simulink model "HighLevel_Example"  (R2024a)
settings: Solver=VariableStepAuto  StartTime=0.0  StopTime=10.0  RelTol=1e-3
settings Model: Creator=Tamir Azaouag  LastModifiedBy=Tamir Azaouag

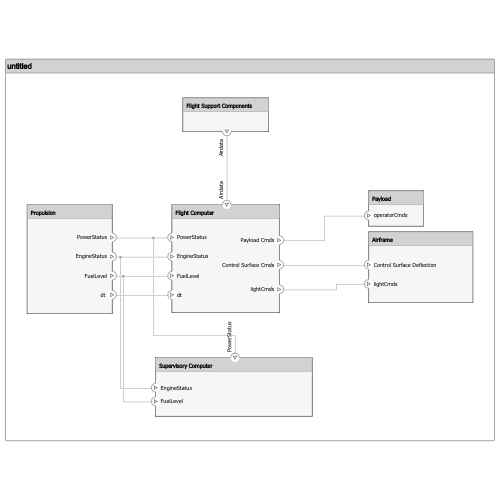
[thumbnail: Simulink's stored preview of the top-level diagram]
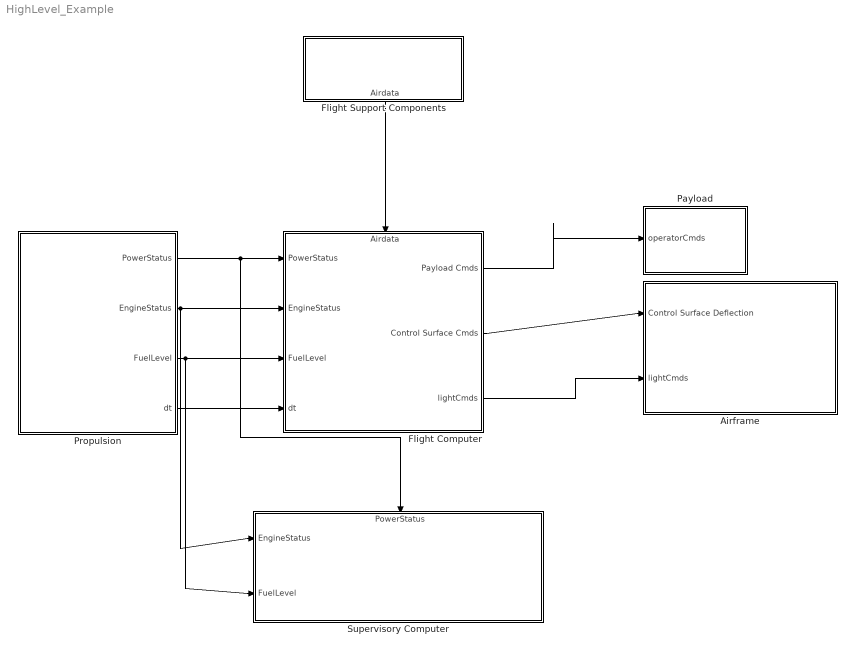
== system HighLevel_Example ==
  Airframe : Subsystem
      settings: PortSchema="{\"entries\":[{\"content\":{\"headerSize\":26,\"margin\":15,\"minimumSpacing\":25,\"sides\":[{\"content\":{\"connectorIds\":[\"In1\",\"In2\"]},\"type\":\"ConnectorPlacement.EquallySpacedRectSide\",\"uuid\":\"2c5e2d04-4906-4331-9418-21fa8db35aaf\"},{\"content\":{\"side\":\"RIGHT\"},\"type\":\"ConnectorPlacement.EquallySpacedRectSide\",\"uuid\":\"94a89f28-0e32-42bb-af58-158d3f1cfd39\"},{\"content\":{\"side\":\"TOP\"},\"type\":\"ConnectorPlacement.EquallySpacedRectSide\",\"uuid\":\"d206ce3f-8f92-44db-9478-82f14b2d4cfb\"}]},\"type\":\"ConnectorPlacement.EquallySpacedConnector\",\"uuid\":\"3d641880-63ee-42e2-927a-a7c9f20600aa\"}],\"packageUris\":[\"http://schema.mathworks.com/mf0/Connector/R2020b\"],\"version\":\"1.0\"}"
  Flight Computer : Subsystem
      settings: PortSchema="{\"entries\":[{\"content\":{\"headerSize\":26,\"margin\":15,\"minimumSpacing\":25,\"sides\":[{\"content\":{\"connectorIds\":[\"In1\",\"In2\",\"In3\",\"In4\"]},\"type\":\"ConnectorPlacement.EquallySpacedRectSide\",\"uuid\":\"2c5e2d04-4906-4331-9418-21fa8db35aaf\"},{\"content\":{\"connectorIds\":[\"Out1\",\"Out2\",\"Out3\"],\"side\":\"RIGHT\"},\"type\":\"ConnectorPlacement.EquallySpacedRectSide\",\"uuid\":\"94a89f28-0e32-42bb-af58-158d3f1cfd39\"},{\"content\":{\"connectorIds\":[\"In5\"],\"side\":\"TOP\"},\"type\":\"ConnectorPlacement.EquallySpacedRectSide\",\"uuid\":\"d206ce3f-8f92-44db-9478-82f14b2d4cfb\"}]},\"type\":\"ConnectorPlacement.EquallySpacedConnector\",\"uuid\":\"3d641880-63ee-42e2-927a-a7c9f20600aa\"}],\"packageUris\":[\"http://schema.mathworks.com/mf0/Connector/R2020b\"],\"version\":\"1.0\"}"
  Flight Support Components : Subsystem
      settings: PortSchema="{\"entries\":[{\"content\":{\"headerSize\":26,\"margin\":15,\"minimumSpacing\":25,\"sides\":[{\"content\":{},\"type\":\"ConnectorPlacement.EquallySpacedRectSide\",\"uuid\":\"2c5e2d04-4906-4331-9418-21fa8db35aaf\"},{\"content\":{\"side\":\"RIGHT\"},\"type\":\"ConnectorPlacement.EquallySpacedRectSide\",\"uuid\":\"94a89f28-0e32-42bb-af58-158d3f1cfd39\"},{\"content\":{\"side\":\"TOP\"},\"type\":\"ConnectorPlacement.EquallySpacedRectSide\",\"uuid\":\"d206ce3f-8f92-44db-9478-82f14b2d4cfb\"},{\"content\":{\"connectorIds\":[\"Out1\"],\"side\":\"BOTTOM\"},\"type\":\"ConnectorPlacement.EquallySpacedRectSide\",\"uuid\":\"ce0da822-1c1c-451b-a130-825bfb22f620\"}]},\"type\":\"ConnectorPlacement.EquallySpacedConnector\",\"uuid\":\"3d641880-63ee-42e2-927a-a7c9f20600aa\"}],\"packageUris\":[\"http://schema.mathworks.com/mf0/Connector/R2020b\"],\"version\":\"1.0\"}"
  "Payload " : Subsystem
      settings: PortSchema="{\"entries\":[{\"content\":{\"headerSize\":26,\"margin\":15,\"minimumSpacing\":25,\"sides\":[{\"content\":{\"connectorIds\":[\"In1\"]},\"type\":\"ConnectorPlacement.EquallySpacedRectSide\",\"uuid\":\"2c5e2d04-4906-4331-9418-21fa8db35aaf\"},{\"content\":{\"side\":\"RIGHT\"},\"type\":\"ConnectorPlacement.EquallySpacedRectSide\",\"uuid\":\"94a89f28-0e32-42bb-af58-158d3f1cfd39\"},{\"content\":{\"side\":\"TOP\"},\"type\":\"ConnectorPlacement.EquallySpacedRectSide\",\"uuid\":\"d206ce3f-8f92-44db-9478-82f14b2d4cfb\"}]},\"type\":\"ConnectorPlacement.EquallySpacedConnector\",\"uuid\":\"3d641880-63ee-42e2-927a-a7c9f20600aa\"}],\"packageUris\":[\"http://schema.mathworks.com/mf0/Connector/R2020b\"],\"version\":\"1.0\"}"
  "Propulsion " : Subsystem
      settings: PortSchema="{\"entries\":[{\"content\":{\"headerSize\":26,\"margin\":15,\"minimumSpacing\":25,\"sides\":[{\"content\":{},\"type\":\"ConnectorPlacement.EquallySpacedRectSide\",\"uuid\":\"2c5e2d04-4906-4331-9418-21fa8db35aaf\"},{\"content\":{\"connectorIds\":[\"Out1\",\"Out2\",\"Out3\",\"Out4\"],\"side\":\"RIGHT\"},\"type\":\"ConnectorPlacement.EquallySpacedRectSide\",\"uuid\":\"94a89f28-0e32-42bb-af58-158d3f1cfd39\"},{\"content\":{\"side\":\"TOP\"},\"type\":\"ConnectorPlacement.EquallySpacedRectSide\",\"uuid\":\"d206ce3f-8f92-44db-9478-82f14b2d4cfb\"}]},\"type\":\"ConnectorPlacement.EquallySpacedConnector\",\"uuid\":\"3d641880-63ee-42e2-927a-a7c9f20600aa\"}],\"packageUris\":[\"http://schema.mathworks.com/mf0/Connector/R2020b\"],\"version\":\"1.0\"}"
  Supervisory Computer : Subsystem
      settings: PortSchema="{\"entries\":[{\"content\":{\"headerSize\":26,\"margin\":15,\"minimumSpacing\":25,\"sides\":[{\"content\":{\"connectorIds\":[\"In1\",\"In2\"]},\"type\":\"ConnectorPlacement.EquallySpacedRectSide\",\"uuid\":\"2c5e2d04-4906-4331-9418-21fa8db35aaf\"},{\"content\":{\"side\":\"RIGHT\"},\"type\":\"ConnectorPlacement.EquallySpacedRectSide\",\"uuid\":\"94a89f28-0e32-42bb-af58-158d3f1cfd39\"},{\"content\":{\"connectorIds\":[\"In3\"],\"side\":\"TOP\"},\"type\":\"ConnectorPlacement.EquallySpacedRectSide\",\"uuid\":\"d206ce3f-8f92-44db-9478-82f14b2d4cfb\"}]},\"type\":\"ConnectorPlacement.EquallySpacedConnector\",\"uuid\":\"3d641880-63ee-42e2-927a-a7c9f20600aa\"}],\"packageUris\":[\"http://schema.mathworks.com/mf0/Connector/R2020b\"],\"version\":\"1.0\"}"
  wires:
  Flight Computer/1(Payload Cmds) -> "Payload "/1(operatorCmds)
  Flight Computer/3(lightCmds) -> Airframe/2(lightCmds)
  Flight Computer/2(Control Surface Cmds) -> Airframe/1(Control Surface Deflection)
  Flight Support Components/1("Airdata ") -> Flight Computer/5("Airdata ")
  "Propulsion "/4("dt ") -> Flight Computer/4("dt ")
  "Propulsion "/2(EngineStatus) -> Flight Computer/2(EngineStatus), Supervisory Computer/1(EngineStatus)
  "Propulsion "/3(FuelLevel) -> Supervisory Computer/2(FuelLevel), Flight Computer/3(FuelLevel)
  "Propulsion "/1(PowerStatus) -> Supervisory Computer/3(PowerStatus), Flight Computer/1(PowerStatus)

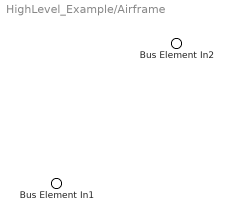
== system HighLevel_Example/Airframe ==
  Bus Element In2 : Inport  PortName=Control Surface Deflection
  Bus Element In1 : Inport  Port=2  PortName=lightCmds

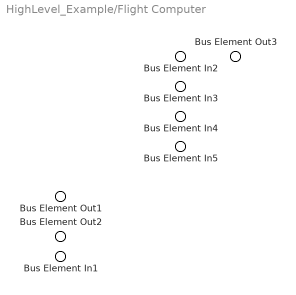
== system HighLevel_Example/Flight Computer ==
  Bus Element In5 : Inport  PortName=PowerStatus
  Bus Element In3 : Inport  Port=2  PortName=EngineStatus
  Bus Element In4 : Inport  Port=3  PortName=FuelLevel
  Bus Element In2 : Inport  Port=4  PortName=dt
  Bus Element In1 : Inport  Port=5  PortName=Airdata
  Bus Element Out1 : Outport  PortName=Payload Cmds
  Bus Element Out3 : Outport  Port=2  PortName=Control Surface Cmds
  Bus Element Out2 : Outport  Port=3  PortName=lightCmds

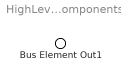
== system HighLevel_Example/Flight Support Components ==
  Bus Element Out1 : Outport  PortName=Airdata

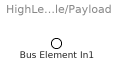
== system HighLevel_Example/Payload  ==
  Bus Element In1 : Inport  PortName=operatorCmds

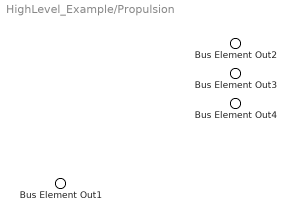
== system HighLevel_Example/Propulsion  ==
  Bus Element Out4 : Outport  PortName=PowerStatus
  Bus Element Out2 : Outport  Port=2  PortName=EngineStatus
  Bus Element Out3 : Outport  Port=3  PortName=FuelLevel
  Bus Element Out1 : Outport  Port=4  PortName=dt

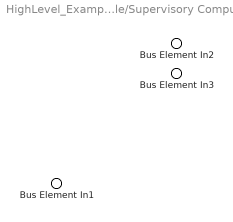
== system HighLevel_Example/Supervisory Computer ==
  Bus Element In3 : Inport  PortName=EngineStatus
  Bus Element In2 : Inport  Port=2  PortName=FuelLevel
  Bus Element In1 : Inport  Port=3  PortName=PowerStatus
